simulink model "BalanceCode_M2V5_Micro"  (R2015a)
settings: Solver=FixedStepDiscrete  SolverMode=SingleTasking  StartTime=0.0  StopTime=inf  FixedStep=TS  RelTol=1e-3
PostLoadFcn:
  | KLQR=[20.0000   13.2675  -28.8721   -1.6327];
  | GS = 1.3316e-04;
  | ES = 0.0047;
  | Rw = 0.022; % radius of wheel in meters
  | KLQRC=KLQR.*[-Rw -Rw 1 1]; % combined LQR Gain with wheel radius scaling
  | TS=.007;tstart=TS*110;
  | LPF=tf(1,[.03 1]);
  | LPFdt=c2d(LPF,TS,'tustin');
  | [num,den] = tfdata(LPFdt);
  | Cnum=num{:};Cden=den{:};
  | disp('controller loaded')
libraries: RASPlib x4, simulink x2, arduinolib x2, MinSegLibrary_M2V5 x2, MinSegLibrary_M1V4 x1
settings Model: FPTRunName=FPA_Reference  SimulationMode=external  ExtModeTrigDuration=2  Creator=Alec  LastModifiedBy=hurstj
settings OptimizationCC: ExpressionDepthLimit=2147483647  OptimizeModelRefInitCode=on  LifeSpan=1
settings DebuggingCC: UnderspecifiedInitializationDetection=Classic  MergeDetectMultiDrivingBlocksExec=none  StateNameClashWarn=warning
settings HardwareCC: ProdBitPerInt=16  ProdBitPerPointer=8  ProdIntDivRoundTo=Zero  ProdEndianess=LittleEndian  ProdWordSize=8  ProdHWDeviceType=Atmel->AVR
settings RTWCC: SystemTargetFile=realtime.tlc  GenerateMakefile=off  TemplateMakefile=realtime.tmf  Description=Real-Time Toolbox  RTWVerbose=off
settings CodeAppCC: CustomSymbolStrType=$N$R$M  InternalIdentifier=Classic
settings ERTTargetCC: CombineOutputUpdateFcns=off  ExtModeTransport=3  ExtModeMexFile=ext_serial_win32_comm_rtt  ExtModeMexArgs=0 97 115200  ERTSrcFileBannerTemplate=realtime_code_template.cgt  ERTHdrFileBannerTemplate=realtime_code_template.cgt  ERTDataSrcFileTemplate=realtime_code_template.cgt  ERTDataHdrFileTemplate=realtime_code_template.cgt  ERTCustomFileTemplate=realtime_file_process.tlc

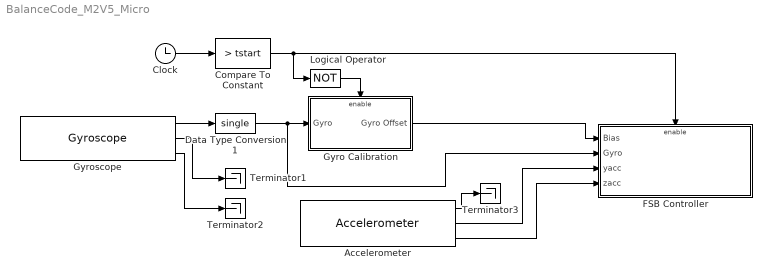
== system BalanceCode_M2V5_Micro ==
  Accelerometer : RASPlib/Accelerometer  SimulateUsing=Code generation
  Clock : Clock
  Compare To Constant : simulink/Logic and Bit Operations/Compare To Constant  relop=>  const=tstart  OutDataTypeStr=boolean
  Data Type Conversion1 : DataTypeConversion  OutDataTypeStr=single
  FSB Controller : Subsystem
  Gyro Calibration : Subsystem  TreatAsAtomicUnit=on
  Gyroscope : RASPlib/Gyroscope  DLPFmode=0
  Logical Operator : Logic  Operator=NOT  AllPortsSameDT=off  OutDataTypeStr=boolean
  Terminator1 : Terminator
  Terminator2 : Terminator
  Terminator3 : Terminator
  wires:
  Clock/1 -> Compare To Constant/1
  Compare To Constant/1 -> Logical Operator/1, FSB Controller/Enable
  Gyro Calibration/1(Gyro Offset) -> FSB Controller/1(Bias)
  Gyroscope/1 -> Data Type Conversion1/1
  Logical Operator/1 -> Gyro Calibration/Enable
  Data Type Conversion1/1 -> FSB Controller/2(Gyro), Gyro Calibration/1(Gyro)
  Accelerometer/2 -> FSB Controller/3("yacc ")
  Accelerometer/3 -> FSB Controller/4("zacc ")
  Gyroscope/2 -> Terminator1/1
  Gyroscope/3 -> Terminator2/1
  Accelerometer/1 -> Terminator3/1

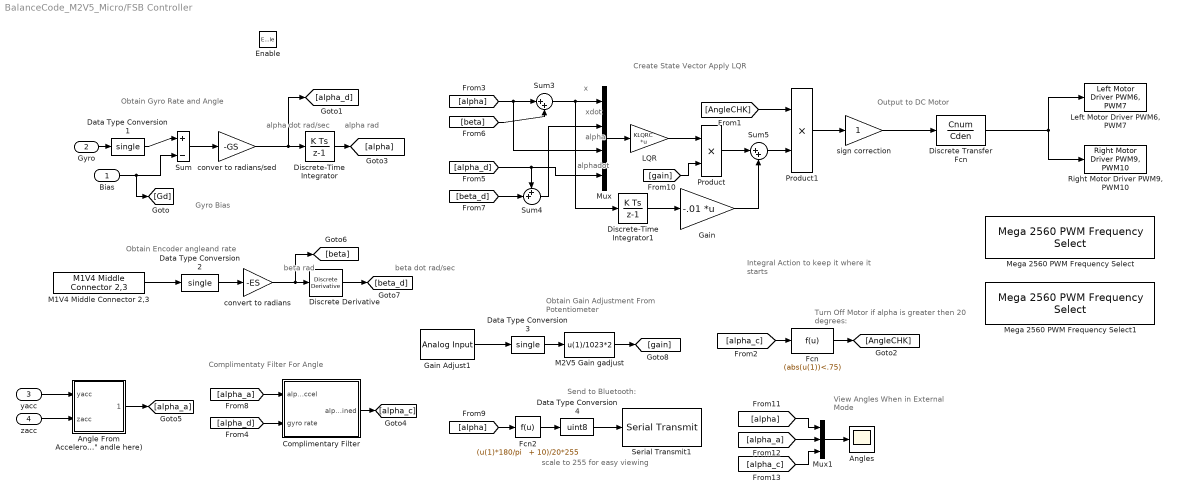
== system BalanceCode_M2V5_Micro/FSB Controller ==
  note: scale to 255 for easy viewing
  note: Integral Action to keep
      |  it where it starts
  note: Gyro
      | Bias
  note: Turn Off Motor if alpha
      | is greater then 20 degrees:
  note: Output to DC Motor
  note: Create State Vector
      | Apply LQR
  note: Obtain Encoder angleand rate
  note: Obtain Gyro Rate and Angle
  note: xdot
  note: x
  note: beta
      | rad
  note: alpha dot
      | rad/sec
  note: alpha
      | rad
  note: beta dot
      | rad/sec
  note: alpha
  note: alphadot
  note: Complimentaty Filter For Angle
  note: Obtain Gain Adjustment
      | From Potentiometer
  note: Send to Bluetooth:
  note: View Angles When in
      | External Mode
  Bias : Inport
  Gyro : Inport  Port=2
  "yacc " : Inport  Port=3
  "zacc " : Inport  Port=4
  Enable : EnablePort
  " Complimentary Filter" : Subsystem
  "Angle From Accelerometer (adjust \"zero\" andle here)" : Subsystem
  Angles : Scope
      settings: YMin=-0.5  YMax=0.6  SaveName=ScopeData2
  Data Type Conversion1 : DataTypeConversion  OutDataTypeStr=single
  Data Type Conversion2 : DataTypeConversion  OutDataTypeStr=single
  Data Type Conversion3 : DataTypeConversion  OutDataTypeStr=single
  Data Type Conversion4 : DataTypeConversion  OutDataTypeStr=uint8
  Discrete Derivative : simulink/Discrete/Discrete Derivative  gainval=1.0  ICPrevScaledInput=0.0  InputProcessing=Inherited  OutMin=[]  OutMax=[]  OutDataType=fixdt(1, 16)  OutScaling=2^-10  DoSatur=off
  Discrete Transfer Fcn : DiscreteTransferFcn  Numerator=Cnum  Denominator=Cden
  Discrete-Time Integrator : DiscreteIntegrator  SampleTime=TS
  Discrete-Time Integrator1 : DiscreteIntegrator  SampleTime=TS
  Fcn : Fcn  Expr=(abs(u(1))<.75)
  Fcn2 : Fcn  Expr="(u(1)*180/pi   + 10)/20*255"
  Gain : Gain  Gain=-.01  Multiplication=Matrix(K*u)
  Gain Adjust1 : arduinolib/Analog Input  pinNumber=0  sampleTime=-1  blockPlatform=arduino
  LQR : Gain  Gain=KLQRC  Multiplication=Matrix(K*u)
  "Left Motor Driver PWM6, PWM7" : MinSegLibrary_M2V5/Left Motor Driver PWM6, PWM7  Vsupply=7.6  PWMoffset=0
  M1V4 Middle Connector 2,3 : MinSegLibrary_M1V4/M1V4 Middle Connector 2,3  Encoder=0  PinA=2  PinB=3
  M2V5 Gain gadjust : Fcn  Expr=u(1)/1023*2
  Mega 2560 PWM Frequency Select : RASPlib/Mega 2560 PWM Frequency Select  Frequency=32KHz  Timer=4 - pins 6, 7, 8
  Mega 2560 PWM Frequency Select1 : RASPlib/Mega 2560 PWM Frequency Select  Frequency=32KHz  Timer=2 - pins 9, 10
  Mux : Mux
  Mux1 : Mux  Inputs=3
  Product : Product  RndMeth=Zero
  Product1 : Product  RndMeth=Zero
  "Right Motor Driver PWM9, PWM10 " : MinSegLibrary_M2V5/Right Motor Driver PWM9, PWM10   Vsupply=7.6  PWMoffset=0
  Serial Transmit1 : arduinolib/Serial Transmit  portNumber=3  blockPlatform=arduino
  Sum : Sum  Inputs=|+-
  Sum3 : Sum  Inputs=|++
  Sum4 : Sum  Inputs=++|
  Sum5 : Sum  Inputs=|++
  conver to radians/sed : Gain  Gain=-GS  OutDataTypeStr=single
  convert to radians : Gain  Gain=-ES  OutDataTypeStr=single
  sign correction : Gain  OutDataTypeStr=single
  wires:
  Sum3/1 -> Mux/1, Discrete-Time Integrator1/1
  Data Type Conversion2/1 -> convert to radians/1
  Bias/1 -> [Gd], Sum/2
  Sum/1 -> conver to radians/sed/1
  Fcn/1 -> [AngleCHK]
  M1V4 Middle Connector 2,3/1 -> Data Type Conversion2/1
  Mux/1 -> LQR/1
  Data Type Conversion1/1 -> Sum/1
  [alpha_c] -> Fcn/1
  conver to radians/sed/1 -> Discrete-Time Integrator/1, [alpha_d]
  Sum4/1 -> Mux/2
  Discrete-Time Integrator/1 -> [alpha]
  Fcn2/1 -> Data Type Conversion4/1
  Data Type Conversion4/1 -> Serial Transmit1/1
  [alpha] -> Sum3/1, Mux/3
  Discrete-Time Integrator1/1 -> Gain/1
  Product/1 -> Sum5/1
  LQR/1 -> Product/1
  Sum5/1 -> Product1/2
  [AngleCHK] -> Product1/1
  Gain/1 -> Sum5/2
  Gyro/1 -> Data Type Conversion1/1
  [alpha_a] -> " Complimentary Filter"/1(alpha accel)
  [alpha_d] -> " Complimentary Filter"/2(gyro rate)
  [alpha_d] -> Mux/4, Sum4/1
  convert to radians/1 -> Discrete Derivative/1, [beta]
  Discrete Derivative/1 -> [beta_d]
  [beta_d] -> Sum4/2
  [beta] -> Sum3/2
  [alpha] -> Fcn2/1
  Data Type Conversion3/1 -> M2V5 Gain gadjust/1
  Gain Adjust1/1 -> Data Type Conversion3/1
  M2V5 Gain gadjust/1 -> [gain]
  [gain] -> Product/2
  [alpha] -> Mux1/1
  [alpha_a] -> Mux1/2
  [alpha_c] -> Mux1/3
  Mux1/1 -> Angles/1
  "yacc "/1 -> "Angle From Accelerometer (adjust \"zero\" andle here)"/1(yacc)
  "zacc "/1 -> "Angle From Accelerometer (adjust \"zero\" andle here)"/2(zacc)
  "Angle From Accelerometer (adjust \"zero\" andle here)"/1(angle rad) -> [alpha_a]
  " Complimentary Filter"/1(alpha combined) -> [alpha_c]
  Product1/1 -> sign correction/1
  sign correction/1 -> Discrete Transfer Fcn/1
  Discrete Transfer Fcn/1 -> "Left Motor Driver PWM6, PWM7"/1, "Right Motor Driver PWM9, PWM10 "/1

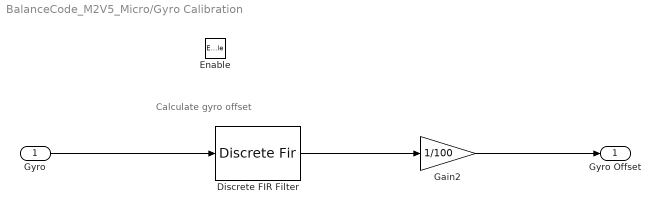
== system BalanceCode_M2V5_Micro/Gyro Calibration ==
  note: Calculate gyro offset
  Gyro : Inport
  Enable : EnablePort
  Discrete FIR Filter : DiscreteFir  Coefficients=ones(1,100)
  Gain2 : Gain  Gain=1/100  OutDataTypeStr=Inherit: Same as input  ParamDataTypeStr=Inherit: Same as input
  Gyro Offset : Outport
  wires:
  Gyro/1 -> Discrete FIR Filter/1
  Discrete FIR Filter/1 -> Gain2/1
  Gain2/1 -> Gyro Offset/1

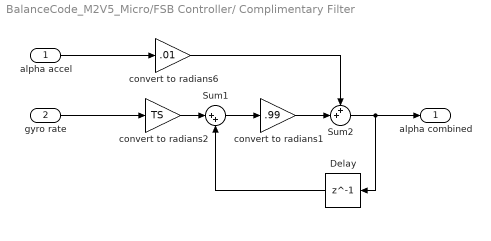
== system BalanceCode_M2V5_Micro/FSB Controller/ Complimentary Filter ==
  alpha accel : Inport
  gyro rate : Inport  Port=2
  Delay : Delay  DelayLength=1  SampleTime=TS
  Sum1 : Sum  Inputs=|++
  Sum2 : Sum  Inputs=++|
  convert to radians1 : Gain  Gain=.99  OutDataTypeStr=single
  convert to radians2 : Gain  Gain=TS  OutDataTypeStr=single
  convert to radians6 : Gain  Gain=.01  OutDataTypeStr=single
  alpha combined : Outport
  wires:
  gyro rate/1 -> convert to radians2/1
  Sum1/1 -> convert to radians1/1
  convert to radians6/1 -> Sum2/1
  alpha accel/1 -> convert to radians6/1
  convert to radians1/1 -> Sum2/2
  Delay/1 -> Sum1/2
  convert to radians2/1 -> Sum1/1
  Sum2/1 -> Delay/1, alpha combined/1

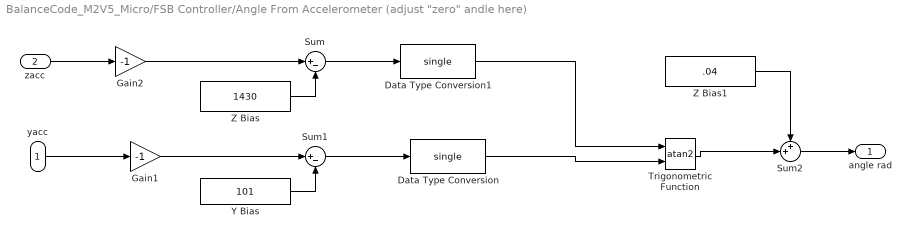
== system BalanceCode_M2V5_Micro/FSB Controller/Angle From Accelerometer (adjust "zero" andle here) ==
  yacc : Inport
  zacc : Inport  Port=2
  Data Type Conversion : DataTypeConversion  OutDataTypeStr=single
  Data Type Conversion1 : DataTypeConversion  OutDataTypeStr=single
  Gain1 : Gain  Gain=-1
  Gain2 : Gain  Gain=-1
  Sum : Sum  Inputs=|+-
  Sum1 : Sum  Inputs=|+-
  Sum2 : Sum  Inputs=++|
  Trigonometric Function : Trigonometry  Operator=atan2
  Y Bias : Constant  Value=101
  Z Bias : Constant  Value=1430
  Z Bias1 : Constant  Value=.04  OutDataTypeStr=single
  angle rad : Outport
  wires:
  Sum1/1 -> Data Type Conversion/1
  Gain2/1 -> Sum/1
  Sum/1 -> Data Type Conversion1/1
  Z Bias/1 -> Sum/2
  Gain1/1 -> Sum1/1
  Y Bias/1 -> Sum1/2
  zacc/1 -> Gain2/1
  yacc/1 -> Gain1/1
  Trigonometric Function/1 -> Sum2/2
  Sum2/1 -> angle rad/1
  Z Bias1/1 -> Sum2/1
  Data Type Conversion1/1 -> Trigonometric Function/1
  Data Type Conversion/1 -> Trigonometric Function/2
